simulink model "CE"  (R2021a)
settings: Solver=VariableStepAuto  StartTime=0.0  StopTime=10.0  RelTol=1e-3
(part 2 of 2)

== stateflow chart CE/Curve/Chart ==
  state off
    en:FunctionConfidenceFlag=0;
    du:FunctionConfidenceFlag=0;
  state on
    state initial
      en:FunctionConfidenceFlag=0;
      du:FunctionConfidenceFlag=0;
    state CE2
      en:FunctionConfidenceFlag=2;
      du:FunctionConfidenceFlag=2;
    state CE3
      en:FunctionConfidenceFlag=3;
      du:FunctionConfidenceFlag=3;
    state CE1
      en:FunctionConfidenceFlag=1;
      du:FunctionConfidenceFlag=1;
    (default) -> initial
    (junction 21) -> initial : [CE2_2_Initial_Condition]
    (junction 27) -> initial : [CE1_2_Initial_Condition]
    CE2 -> (junction 21) [order 2]
    CE1 -> (junction 27) [order 2]
    initial -> (junction 28) [order 3] : [Initial2CE1_Condition]
    initial -> (junction 23) [order 2] : [Initial2CE2_Condition]
    (junction 28) -> CE1
    (junction 23) -> CE2
    initial -> CE3 [order 1] : [Initial2CE3_Condition]
    CE3 -> initial [order 1] : [CE3_2_Initial_Condition]
    CE2 -> CE3 [order 1] : [CE2_2_CE3_Condition]
    CE3 -> CE1 [order 2] : [CE3_2_CE1_Condition]
    CE1 -> CE3 [order 1] : [CE1_2_CE3_Condition]
    CE3 -> CE2 [order 3] : [CE3_2_CE2_Condition]
    CE1 -> (junction 39) [order 3]
    (junction 38) -> CE1
    CE2 -> (junction 36) [order 3]
    (junction 33) -> CE2
    (junction 39) -> (junction 33) : [CE1_2_CE2_Condition]
    (junction 36) -> (junction 38) : [CE2_2_CE1_Condition]
  (default) -> off
  off -> on : [ON2OFF_Condition]
  on -> off : [OFF2ON_Condition]
  data: CE1_2_CE2_Condition input; CE1_2_Initial_Condition input; CE1_2_CE3_Condition input; CE2_2_CE3_Condition input; CE2_2_CE1_Condition input; CE2_2_Initial_Condition input; CE3_2_CE1_Condition input; CE3_2_CE2_Condition input; CE3_2_Initial_Condition input; Initial2CE1_Condition input; Initial2CE2_Condition input; Initial2CE3_Condition input; OFF2ON_Condition input; ON2OFF_Condition input; FunctionConfidenceFlag output

== stateflow chart CE/CruiseOnLane/Chart ==
  state off
    en:FunctionConfidenceFlag=0;
    du:FunctionConfidenceFlag=0;
  state on
    state initial
      en:FunctionConfidenceFlag=0;
      du:FunctionConfidenceFlag=0;
    state CE2
      en:FunctionConfidenceFlag=2;
      du:FunctionConfidenceFlag=2;
    state CE3
      en:FunctionConfidenceFlag=3;
      du:FunctionConfidenceFlag=3;
    state CE1
      en:FunctionConfidenceFlag=1;
      du:FunctionConfidenceFlag=1;
    (default) -> initial
    (junction 21) -> initial : [CE2_2_Initial_Condition]
    (junction 27) -> initial : [CE1_2_Initial_Condition]
    CE2 -> (junction 21) [order 2]
    CE1 -> (junction 27) [order 2]
    initial -> (junction 28) [order 3] : [Initial2CE1_Condition]
    initial -> (junction 23) [order 2] : [Initial2CE2_Condition]
    (junction 28) -> CE1
    (junction 23) -> CE2
    initial -> CE3 [order 1] : [Initial2CE3_Condition]
    CE3 -> initial [order 1] : [CE3_2_Initial_Condition]
    CE2 -> CE3 [order 1] : [CE2_2_CE3_Condition]
    CE3 -> CE1 [order 2] : [CE3_2_CE1_Condition]
    CE1 -> CE3 [order 1] : [CE1_2_CE3_Condition]
    CE3 -> CE2 [order 3] : [CE3_2_CE2_Condition]
    CE1 -> (junction 39) [order 3]
    (junction 38) -> CE1
    CE2 -> (junction 36) [order 3]
    (junction 33) -> CE2
    (junction 39) -> (junction 33) : [CE1_2_CE2_Condition]
    (junction 36) -> (junction 38) : [CE2_2_CE1_Condition]
  (default) -> off
  off -> on : [ON2OFF_Condition]
  on -> off : [OFF2ON_Condition]
  data: CE1_2_CE2_Condition input; CE1_2_Initial_Condition input; CE1_2_CE3_Condition input; CE2_2_CE3_Condition input; CE2_2_CE1_Condition input; CE2_2_Initial_Condition input; CE3_2_CE1_Condition input; CE3_2_CE2_Condition input; CE3_2_Initial_Condition input; Initial2CE1_Condition input; Initial2CE2_Condition input; Initial2CE3_Condition input; OFF2ON_Condition input; ON2OFF_Condition input; FunctionConfidenceFlag output

== stateflow chart CE/Ramp/Chart ==
  state off
    en:FunctionConfidenceFlag=0;
    du:FunctionConfidenceFlag=0;
  state on
    state initial
      en:FunctionConfidenceFlag=0;
      du:FunctionConfidenceFlag=0;
    state CE2
      en:FunctionConfidenceFlag=2;
      du:FunctionConfidenceFlag=2;
    state CE3
      en:FunctionConfidenceFlag=3;
      du:FunctionConfidenceFlag=3;
    state CE1
      en:FunctionConfidenceFlag=1;
      du:FunctionConfidenceFlag=1;
    (default) -> initial
    (junction 21) -> initial : [CE2_2_Initial_Condition]
    (junction 27) -> initial : [CE1_2_Initial_Condition]
    CE2 -> (junction 21) [order 2]
    CE1 -> (junction 27) [order 2]
    initial -> (junction 28) [order 3] : [Initial2CE1_Condition]
    initial -> (junction 23) [order 2] : [Initial2CE2_Condition]
    (junction 28) -> CE1
    (junction 23) -> CE2
    initial -> CE3 [order 1] : [Initial2CE3_Condition]
    CE3 -> initial [order 1] : [CE3_2_Initial_Condition]
    CE2 -> CE3 [order 1] : [CE2_2_CE3_Condition]
    CE3 -> CE1 [order 2] : [CE3_2_CE1_Condition]
    CE1 -> CE3 [order 1] : [CE1_2_CE3_Condition]
    CE3 -> CE2 [order 3] : [CE3_2_CE2_Condition]
    CE1 -> (junction 39) [order 3]
    (junction 38) -> CE1
    CE2 -> (junction 36) [order 3]
    (junction 33) -> CE2
    (junction 39) -> (junction 33) : [CE1_2_CE2_Condition]
    (junction 36) -> (junction 38) : [CE2_2_CE1_Condition]
  (default) -> off
  off -> on : [ON2OFF_Condition]
  on -> off : [OFF2ON_Condition]
  data: CE1_2_CE2_Condition input; CE1_2_Initial_Condition input; CE1_2_CE3_Condition input; CE2_2_CE3_Condition input; CE2_2_CE1_Condition input; CE2_2_Initial_Condition input; CE3_2_CE1_Condition input; CE3_2_CE2_Condition input; CE3_2_Initial_Condition input; Initial2CE1_Condition input; Initial2CE2_Condition input; Initial2CE3_Condition input; OFF2ON_Condition input; ON2OFF_Condition input; FunctionConfidenceFlag output

== stateflow chart CE/Split/Chart ==
  state off
    en:FunctionConfidenceFlag=0;
    du:FunctionConfidenceFlag=0;
  state on
    state initial
      en:FunctionConfidenceFlag=0;
      du:FunctionConfidenceFlag=0;
    state CE2
      en:FunctionConfidenceFlag=2;
      du:FunctionConfidenceFlag=2;
    state CE3
      en:FunctionConfidenceFlag=3;
      du:FunctionConfidenceFlag=3;
    state CE1
      en:FunctionConfidenceFlag=1;
      du:FunctionConfidenceFlag=1;
    (default) -> initial
    (junction 21) -> initial : [CE2_2_Initial_Condition]
    (junction 27) -> initial : [CE1_2_Initial_Condition]
    CE2 -> (junction 21) [order 2]
    CE1 -> (junction 27) [order 2]
    initial -> (junction 28) [order 3] : [Initial2CE1_Condition]
    initial -> (junction 23) [order 2] : [Initial2CE2_Condition]
    (junction 28) -> CE1
    (junction 23) -> CE2
    initial -> CE3 [order 1] : [Initial2CE3_Condition]
    CE3 -> initial [order 1] : [CE3_2_Initial_Condition]
    CE2 -> CE3 [order 1] : [CE2_2_CE3_Condition]
    CE3 -> CE1 [order 2] : [CE3_2_CE1_Condition]
    CE1 -> CE3 [order 1] : [CE1_2_CE3_Condition]
    CE3 -> CE2 [order 3] : [CE3_2_CE2_Condition]
    CE1 -> (junction 39) [order 3]
    (junction 38) -> CE1
    CE2 -> (junction 36) [order 3]
    (junction 33) -> CE2
    (junction 39) -> (junction 33) : [CE1_2_CE2_Condition]
    (junction 36) -> (junction 38) : [CE2_2_CE1_Condition]
  (default) -> off
  off -> on : [ON2OFF_Condition]
  on -> off : [OFF2ON_Condition]
  data: CE1_2_CE2_Condition input; CE1_2_Initial_Condition input; CE1_2_CE3_Condition input; CE2_2_CE3_Condition input; CE2_2_CE1_Condition input; CE2_2_Initial_Condition input; CE3_2_CE1_Condition input; CE3_2_CE2_Condition input; CE3_2_Initial_Condition input; Initial2CE1_Condition input; Initial2CE2_Condition input; Initial2CE3_Condition input; OFF2ON_Condition input; ON2OFF_Condition input; FunctionConfidenceFlag output

== stateflow chart CE/Construction1/Chart ==
  state off
    en:FunctionConfidenceFlag=0;
    du:FunctionConfidenceFlag=0;
  state on
    state initial
      en:FunctionConfidenceFlag=0;
      du:FunctionConfidenceFlag=0;
    state CE2
      en:FunctionConfidenceFlag=2;
      du:FunctionConfidenceFlag=2;
    state CE3
      en:FunctionConfidenceFlag=3;
      du:FunctionConfidenceFlag=3;
    state CE1
      en:FunctionConfidenceFlag=1;
      du:FunctionConfidenceFlag=1;
    (default) -> initial
    (junction 21) -> initial : [CE2_2_Initial_Condition]
    (junction 27) -> initial : [CE1_2_Initial_Condition]
    CE2 -> (junction 21) [order 2]
    CE1 -> (junction 27) [order 2]
    initial -> (junction 28) [order 3] : [Initial2CE1_Condition]
    initial -> (junction 23) [order 2] : [Initial2CE2_Condition]
    (junction 28) -> CE1
    (junction 23) -> CE2
    initial -> CE3 [order 1] : [Initial2CE3_Condition]
    CE3 -> initial [order 1] : [CE3_2_Initial_Condition]
    CE2 -> CE3 [order 1] : [CE2_2_CE3_Condition]
    CE3 -> CE1 [order 2] : [CE3_2_CE1_Condition]
    CE1 -> CE3 [order 1] : [CE1_2_CE3_Condition]
    CE3 -> CE2 [order 3] : [CE3_2_CE2_Condition]
    CE1 -> (junction 39) [order 3]
    (junction 38) -> CE1
    CE2 -> (junction 36) [order 3]
    (junction 33) -> CE2
    (junction 39) -> (junction 33) : [CE1_2_CE2_Condition]
    (junction 36) -> (junction 38) : [CE2_2_CE1_Condition]
  (default) -> off
  off -> on : [ON2OFF_Condition]
  on -> off : [OFF2ON_Condition]
  data: CE1_2_CE2_Condition input; CE1_2_Initial_Condition input; CE1_2_CE3_Condition input; CE2_2_CE3_Condition input; CE2_2_CE1_Condition input; CE2_2_Initial_Condition input; CE3_2_CE1_Condition input; CE3_2_CE2_Condition input; CE3_2_Initial_Condition input; Initial2CE1_Condition input; Initial2CE2_Condition input; Initial2CE3_Condition input; OFF2ON_Condition input; ON2OFF_Condition input; FunctionConfidenceFlag output

== stateflow chart CE/ILC/Chart ==
  state off
    en:FunctionConfidenceFlag=0;
    du:FunctionConfidenceFlag=0;
  state on
    state initial
      en:FunctionConfidenceFlag=0;
      du:FunctionConfidenceFlag=0;
    state CE2
      en:FunctionConfidenceFlag=2;
      du:FunctionConfidenceFlag=2;
    state CE3
      en:FunctionConfidenceFlag=3;
      du:FunctionConfidenceFlag=3;
    state CE1
      en:FunctionConfidenceFlag=1;
      du:FunctionConfidenceFlag=1;
    (default) -> initial
    (junction 21) -> initial : [CE2_2_Initial_Condition]
    (junction 27) -> initial : [CE1_2_Initial_Condition]
    CE2 -> (junction 21) [order 2]
    CE1 -> (junction 27) [order 2]
    initial -> (junction 28) [order 3] : [Initial2CE1_Condition]
    initial -> (junction 23) [order 2] : [Initial2CE2_Condition]
    (junction 28) -> CE1
    (junction 23) -> CE2
    initial -> CE3 [order 1] : [Initial2CE3_Condition]
    CE3 -> initial [order 1] : [CE3_2_Initial_Condition]
    CE2 -> CE3 [order 1] : [CE2_2_CE3_Condition]
    CE3 -> CE1 [order 2] : [CE3_2_CE1_Condition]
    CE1 -> CE3 [order 1] : [CE1_2_CE3_Condition]
    CE3 -> CE2 [order 3] : [CE3_2_CE2_Condition]
    CE1 -> (junction 39) [order 3]
    (junction 38) -> CE1
    CE2 -> (junction 36) [order 3]
    (junction 33) -> CE2
    (junction 39) -> (junction 33) : [CE1_2_CE2_Condition]
    (junction 36) -> (junction 38) : [CE2_2_CE1_Condition]
  (default) -> off
  off -> on : [ON2OFF_Condition]
  on -> off : [OFF2ON_Condition]
  data: CE1_2_CE2_Condition input; CE1_2_Initial_Condition input; CE1_2_CE3_Condition input; CE2_2_CE3_Condition input; CE2_2_CE1_Condition input; CE2_2_Initial_Condition input; CE3_2_CE1_Condition input; CE3_2_CE2_Condition input; CE3_2_Initial_Condition input; Initial2CE1_Condition input; Initial2CE2_Condition input; Initial2CE3_Condition input; OFF2ON_Condition input; ON2OFF_Condition input; FunctionConfidenceFlag output

== stateflow chart CE/Tunnel/Chart ==
  state off
    en:FunctionConfidenceFlag=0;
    du:FunctionConfidenceFlag=0;
  state on
    state initial
      en:FunctionConfidenceFlag=0;
      du:FunctionConfidenceFlag=0;
    state CE2
      en:FunctionConfidenceFlag=2;
      du:FunctionConfidenceFlag=2;
    state CE3
      en:FunctionConfidenceFlag=3;
      du:FunctionConfidenceFlag=3;
    state CE1
      en:FunctionConfidenceFlag=1;
      du:FunctionConfidenceFlag=1;
    (default) -> initial
    (junction 21) -> initial : [CE2_2_Initial_Condition]
    (junction 27) -> initial : [CE1_2_Initial_Condition]
    CE2 -> (junction 21) [order 2]
    CE1 -> (junction 27) [order 2]
    initial -> (junction 28) [order 3] : [Initial2CE1_Condition]
    initial -> (junction 23) [order 2] : [Initial2CE2_Condition]
    (junction 28) -> CE1
    (junction 23) -> CE2
    initial -> CE3 [order 1] : [Initial2CE3_Condition]
    CE3 -> initial [order 1] : [CE3_2_Initial_Condition]
    CE2 -> CE3 [order 1] : [CE2_2_CE3_Condition]
    CE3 -> CE1 [order 2] : [CE3_2_CE1_Condition]
    CE1 -> CE3 [order 1] : [CE1_2_CE3_Condition]
    CE3 -> CE2 [order 3] : [CE3_2_CE2_Condition]
    CE1 -> (junction 39) [order 3]
    (junction 38) -> CE1
    CE2 -> (junction 36) [order 3]
    (junction 33) -> CE2
    (junction 39) -> (junction 33) : [CE1_2_CE2_Condition]
    (junction 36) -> (junction 38) : [CE2_2_CE1_Condition]
  (default) -> off
  off -> on : [ON2OFF_Condition]
  on -> off : [OFF2ON_Condition]
  data: CE1_2_CE2_Condition input; CE1_2_Initial_Condition input; CE1_2_CE3_Condition input; CE2_2_CE3_Condition input; CE2_2_CE1_Condition input; CE2_2_Initial_Condition input; CE3_2_CE1_Condition input; CE3_2_CE2_Condition input; CE3_2_Initial_Condition input; Initial2CE1_Condition input; Initial2CE2_Condition input; Initial2CE3_Condition input; OFF2ON_Condition input; ON2OFF_Condition input; FunctionConfidenceFlag output

== stateflow chart CE/Construction/Chart ==
  state off
    en:FunctionConfidenceFlag=0;
    du:FunctionConfidenceFlag=0;
  state on
    state initial
      en:FunctionConfidenceFlag=0;
      du:FunctionConfidenceFlag=0;
    state CE2
      en:FunctionConfidenceFlag=2;
      du:FunctionConfidenceFlag=2;
    state CE3
      en:FunctionConfidenceFlag=3;
      du:FunctionConfidenceFlag=3;
    state CE1
      en:FunctionConfidenceFlag=1;
      du:FunctionConfidenceFlag=1;
    (default) -> initial
    (junction 21) -> initial : [CE2_2_Initial_Condition]
    (junction 27) -> initial : [CE1_2_Initial_Condition]
    CE2 -> (junction 21) [order 2]
    CE1 -> (junction 27) [order 2]
    initial -> (junction 28) [order 3] : [Initial2CE1_Condition]
    initial -> (junction 23) [order 2] : [Initial2CE2_Condition]
    (junction 28) -> CE1
    (junction 23) -> CE2
    initial -> CE3 [order 1] : [Initial2CE3_Condition]
    CE3 -> initial [order 1] : [CE3_2_Initial_Condition]
    CE2 -> CE3 [order 1] : [CE2_2_CE3_Condition]
    CE3 -> CE1 [order 2] : [CE3_2_CE1_Condition]
    CE1 -> CE3 [order 1] : [CE1_2_CE3_Condition]
    CE3 -> CE2 [order 3] : [CE3_2_CE2_Condition]
    CE1 -> (junction 39) [order 3]
    (junction 38) -> CE1
    CE2 -> (junction 36) [order 3]
    (junction 33) -> CE2
    (junction 39) -> (junction 33) : [CE1_2_CE2_Condition]
    (junction 36) -> (junction 38) : [CE2_2_CE1_Condition]
  (default) -> off
  off -> on : [ON2OFF_Condition]
  on -> off : [OFF2ON_Condition]
  data: CE1_2_CE2_Condition input; CE1_2_Initial_Condition input; CE1_2_CE3_Condition input; CE2_2_CE3_Condition input; CE2_2_CE1_Condition input; CE2_2_Initial_Condition input; CE3_2_CE1_Condition input; CE3_2_CE2_Condition input; CE3_2_Initial_Condition input; Initial2CE1_Condition input; Initial2CE2_Condition input; Initial2CE3_Condition input; OFF2ON_Condition input; ON2OFF_Condition input; FunctionConfidenceFlag output

== stateflow chart CE/TrafficDencity/Chart ==
  (default) -> (junction 3) : {TrafficDencity=0;
      | j=1;
      | counter=0;}
  (junction 3) -> (junction 5) [order 1] : [j<49;]
  (junction 5) -> (junction 10) [order 1] : [(SDF_Object.dx<=50||SDF_Object.d>=-30)...
      | &&SDF_Object.dy<=13]
  (junction 7) -> (junction 3) : {j = j + 1;}
  (junction 3) -> (junction 17) [order 2]
  (junction 5) -> (junction 7) [order 2]
  (junction 10) -> (junction 14) : {counter = counter + 1}
  (junction 14) -> (junction 7)
  (junction 17) -> (junction 19) [order 1] : [counter>=5]
  (junction 19) -> (junction 31) [order 2] : [counter<=10]
  (junction 17) -> (junction 27) [order 2] : {TrafficDencity=1}
  (junction 19) -> (junction 21) [order 1] : {TrafficDencity=2}
  (junction 31) -> (junction 33) : {TrafficDencity=1}
  (junction 21) -> (junction 27)
  (junction 33) -> (junction 21)
  (junction 27) -> (junction 37)
  data: counter local; j local; TrafficDencity output; SDF_Object input

== stateflow chart CE/CutinObjDengerCal/CutinTargetSearch ==
  (default) -> (junction 64)
  (junction 64) -> (junction 65) : {j=1;
      | CutinTarget.dX=999;
      | CutinTarget.dy=999;}
  (junction 65) -> (junction 66) [order 1] : [j<=50]
  (junction 66) -> (junction 67) [order 1] : [SDF_Object(j).ID==CutinTarget_ID]
  (junction 70) -> (junction 65)
  (junction 65) -> (junction 69) [order 2] : {CutinTarget=OBJ_VD_ZERO;}
  (junction 66) -> (junction 70) [order 2] : {j=j+1;}
  (junction 67) -> (junction 68) : {CutinTarget.dX=SDF_Object(j).dx;
      | CutinTarget.dy=SDF_Object(j).dy;}
  data: j local; OBJ_VD_ZERO input Bus: gSDF_stObjects_Type; CutinTarget_ID input; SDF_Object input; CutinTarget output

== stateflow chart CE/LaneChange/Chart ==
  state off
    en:FunctionConfidenceFlag=0;
    du:FunctionConfidenceFlag=0;
  state on
    state initial
      en:FunctionConfidenceFlag=0;
      du:FunctionConfidenceFlag=0;
    state CE2
      en:FunctionConfidenceFlag=2;
      du:FunctionConfidenceFlag=2;
    state CE3
      en:FunctionConfidenceFlag=3;
      du:FunctionConfidenceFlag=3;
    state CE1
      en:FunctionConfidenceFlag=1;
      du:FunctionConfidenceFlag=1;
    (default) -> initial
    (junction 21) -> initial : [CE2_2_Initial_Condition]
    (junction 27) -> initial : [CE1_2_Initial_Condition]
    CE2 -> (junction 21) [order 2]
    CE1 -> (junction 27) [order 2]
    initial -> (junction 28) [order 3] : [Initial2CE1_Condition]
    initial -> (junction 23) [order 2] : [Initial2CE2_Condition]
    (junction 28) -> CE1
    (junction 23) -> CE2
    initial -> CE3 [order 1] : [Initial2CE3_Condition]
    CE3 -> initial [order 1] : [CE3_2_Initial_Condition]
    CE2 -> CE3 [order 1] : [CE2_2_CE3_Condition]
    CE3 -> CE1 [order 2] : [CE3_2_CE1_Condition]
    CE1 -> CE3 [order 1] : [CE1_2_CE3_Condition]
    CE3 -> CE2 [order 3] : [CE3_2_CE2_Condition]
    CE1 -> (junction 39) [order 3]
    (junction 38) -> CE1
    CE2 -> (junction 36) [order 3]
    (junction 33) -> CE2
    (junction 39) -> (junction 33) : [CE1_2_CE2_Condition]
    (junction 36) -> (junction 38) : [CE2_2_CE1_Condition]
  (default) -> off
  off -> on : [ON2OFF_Condition]
  on -> off : [OFF2ON_Condition]
  data: CE1_2_CE2_Condition input; CE1_2_Initial_Condition input; CE1_2_CE3_Condition input; CE2_2_CE3_Condition input; CE2_2_CE1_Condition input; CE2_2_Initial_Condition input; CE3_2_CE1_Condition input; CE3_2_CE2_Condition input; CE3_2_Initial_Condition input; Initial2CE1_Condition input; Initial2CE2_Condition input; Initial2CE3_Condition input; OFF2ON_Condition input; ON2OFF_Condition input; FunctionConfidenceFlag output
